simulink model "Point_4"  (R2024b)
settings: Solver=VariableStepAuto  StartTime=0.0  StopTime=15  RelTol=1e-3
libraries: robotmobilelib x1
settings Model: Creator=emanuela  LastModifiedBy=emanuela
settings DataIOCC: SaveFormat=Array

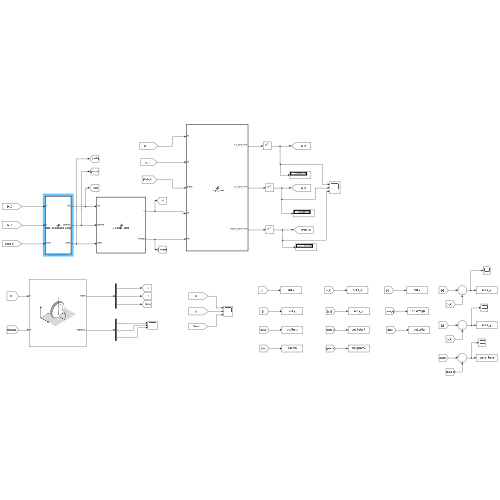
[thumbnail: Simulink's stored preview of the top-level diagram]
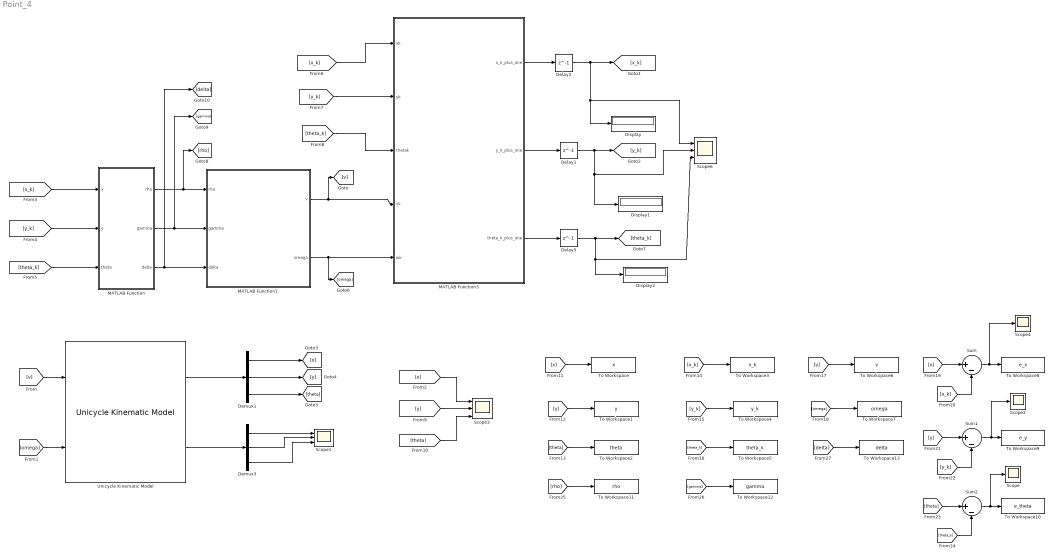
== system Point_4 ==
  Delay1 : Delay  DelayLength=1  InitialCondition=1  SampleTime=0.01
  Delay2 : Delay  DelayLength=1  InitialCondition=5  SampleTime=0.01
  Delay5 : Delay  DelayLength=1  InitialCondition=pi/4  SampleTime=0.01
  Demux1 : Demux  Outputs=3
  Demux3 : Demux  Outputs=3
  Display : Display
  Display1 : Display
  Display2 : Display
  MATLAB Function : MATLAB Function  TreatAsAtomicUnit=on
  MATLAB Function1 : MATLAB Function  TreatAsAtomicUnit=on
  MATLAB Function3 : MATLAB Function  TreatAsAtomicUnit=on
  Scope : Scope
  Scope1 : Scope  NumInputPorts=3
  Scope2 : Scope
  Scope3 : Scope  NumInputPorts=3
  Scope4 : Scope
  Scope6 : Scope  NumInputPorts=3
  Sum : Sum  Inputs=|+-
  Sum1 : Sum  Inputs=|+-
  Sum2 : Sum  Inputs=|+-
  To Workspace : ToWorkspace  VariableName=x  SaveFormat=Structure With Time  SampleTime=-1
  To Workspace1 : ToWorkspace  VariableName=y  SaveFormat=Structure With Time  SampleTime=-1
  To Workspace10 : ToWorkspace  VariableName=e_theta  SaveFormat=Structure With Time  SampleTime=-1
  To Workspace11 : ToWorkspace  VariableName=rho  SaveFormat=Structure With Time  SampleTime=-1
  To Workspace12 : ToWorkspace  VariableName=gamma  SaveFormat=Structure With Time  SampleTime=-1
  To Workspace13 : ToWorkspace  VariableName=delta  SaveFormat=Structure With Time  SampleTime=-1
  To Workspace2 : ToWorkspace  VariableName=theta  SaveFormat=Structure With Time  SampleTime=-1
  To Workspace3 : ToWorkspace  VariableName=x_k  SaveFormat=Structure With Time  SampleTime=-1
  To Workspace4 : ToWorkspace  VariableName=y_k  SaveFormat=Structure With Time  SampleTime=-1
  To Workspace5 : ToWorkspace  VariableName=theta_k  SaveFormat=Structure With Time  SampleTime=-1
  To Workspace6 : ToWorkspace  VariableName=v  SaveFormat=Structure With Time  SampleTime=-1
  To Workspace7 : ToWorkspace  VariableName=omega  SaveFormat=Structure With Time  SampleTime=-1
  To Workspace8 : ToWorkspace  VariableName=e_x  SaveFormat=Structure With Time  SampleTime=-1
  To Workspace9 : ToWorkspace  VariableName=e_y  SaveFormat=Structure With Time  SampleTime=-1
  Unicycle Kinematic Model : robotmobilelib/Unicycle Kinematic Model  VehicleInputs=Vehicle Speed & Heading Angular Velocity  WheelRadius=0.1  WheelSpeedRange=[-Inf Inf]  InitialState=[5; 1; pi/4]  SimulateUsing=Interpreted execution
  wires:
  MATLAB Function/3(delta) -> [delta], MATLAB Function1/3(delta)
  [theta_k] -> MATLAB Function/3(theta)
  MATLAB Function/2(gamma) -> [gamma], MATLAB Function1/2(gamma)
  [y_k] -> MATLAB Function/2(y)
  MATLAB Function/1(rho) -> MATLAB Function1/1(rho), [rho]
  [x_k] -> MATLAB Function/1(x)
  Delay5/1 -> Display2/1, Scope6/3, [theta_k]
  [x_k] -> MATLAB Function3/1(xk)
  MATLAB Function3/3(theta_k_plus_one) -> Delay5/1
  [y_k] -> MATLAB Function3/2(yk)
  [theta_k] -> MATLAB Function3/3(thetak)
  Delay2/1 -> Display/1, Scope6/1, [x_k]
  Delay1/1 -> Scope6/2, Display1/1, [y_k]
  MATLAB Function3/1(x_k_plus_one) -> Delay2/1
  MATLAB Function3/2(y_k_plus_one) -> Delay1/1
  MATLAB Function1/2(omega) -> MATLAB Function3/5(wk), [omega]
  MATLAB Function1/1(v) -> [v], MATLAB Function3/4(vk)
  Unicycle Kinematic Model/1 -> Demux1/1
  Unicycle Kinematic Model/2 -> Demux3/1
  Demux1/1 -> [x]
  Demux3/1 -> Scope1/1
  Demux1/2 -> [y]
  Demux1/3 -> [theta]
  Demux3/3 -> Scope1/3
  Demux3/2 -> Scope1/2
  [v] -> Unicycle Kinematic Model/1
  [omega] -> Unicycle Kinematic Model/2
  [x] -> Scope3/1
  [y] -> Scope3/2
  [theta] -> Scope3/3
  [theta] -> To Workspace2/1
  [y] -> To Workspace1/1
  [x] -> To Workspace/1
  [theta_k] -> To Workspace5/1
  [y_k] -> To Workspace4/1
  [x_k] -> To Workspace3/1
  [omega] -> To Workspace7/1
  [v] -> To Workspace6/1
  [x] -> Sum/1
  [x_k] -> Sum/2
  Sum/1 -> Scope4/1, To Workspace8/1
  Sum1/1 -> Scope2/1, To Workspace9/1
  [y] -> Sum1/1
  [y_k] -> Sum1/2
  [theta_k] -> Sum2/2
  [theta] -> Sum2/1
  Sum2/1 -> Scope/1, To Workspace10/1
  [delta] -> To Workspace13/1
  [rho] -> To Workspace11/1
  [gamma] -> To Workspace12/1

== matlab function Point_4/MATLAB Function1 ==
  data: rho input; v output; gamma input; delta input; omega output
function [v,omega] = v_omega_comp(rho,gamma,delta)

% k1 = 0.5;
% k2 = 1.6;
% k3 = 2.2;

k1 = 2;   
k2 = 4;  
k3 = 0.8;   

v = k1*rho*cos(gamma);

omega = k2*gamma+k1*sin(gamma)*cos(gamma)*(1+k3*(delta/gamma));

end

== matlab function Point_4/MATLAB Function ==
  data: x input; rho output; y input; theta input; gamma output; delta output
function  [rho, gamma,delta] = polar_coordinates_comp(x, y, theta)

rho = sqrt(x^2 + y^2);

gamma = atan2(y,x)-theta+pi;

delta = gamma+theta;

end

== matlab function Point_4/MATLAB Function3 ==
  data: xk input; x_k_plus_one output; yk input; thetak input; vk input; wk input; y_k_plus_one output; theta_k_plus_one output
function [x_k_plus_one, y_k_plus_one,theta_k_plus_one] = Runge_Kutta(xk,yk,thetak, vk, wk)

Ts = 0.01;

x_k_plus_one = xk + vk*Ts*cos(thetak + (wk*Ts)/2);

y_k_plus_one = yk + vk*Ts*sin(thetak + (wk*Ts)/2);

theta_k_plus_one = thetak + (wk*Ts);

end
